simulink model "temp_gearSelector"  (R2020a)
settings: Solver=VariableStepAuto  StartTime=0.0  StopTime=10.0  RelTol=1e-3
settings Model: Creator=rosswilkinson  LastModifiedBy=rosswilkinson

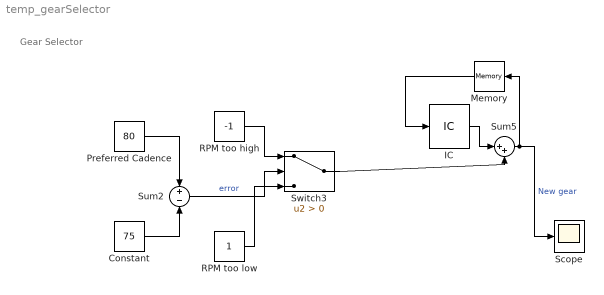
== system temp_gearSelector ==
  note: Gear Selector
  Constant : Constant  Value=75
  IC : InitialCondition  Value=16
  Memory : Memory
  Preferred Cadence : Constant  Value=80
  RPM too high : Constant  Value=-1
  RPM too low : Constant
  Scope : Scope
  Sum2 : Sum  Inputs=+-
  Sum5 : Sum  Inputs=|++
  Switch3 : Switch  Criteria=u2 > Threshold
  wires:
  Switch3/1 -> Sum5/2
  Constant/1 -> Sum2/2
  Sum5/1 -> Memory/1, Scope/1  "New gear"
  Preferred Cadence/1 -> Sum2/1
  RPM too low/1 -> Switch3/3
  RPM too high/1 -> Switch3/1
  Sum2/1 -> Switch3/2  "error"
  IC/1 -> Sum5/1
  Memory/1 -> IC/1
